simulink model "force_control_sim"  (R2013a)
settings: Solver=FixedStepDiscrete  StartTime=0.0  StopTime=10  FixedStep=.001  RelTol=1e-3
settings Model: Creator=dholley  LastModifiedBy=dholley
settings DataIOCC: LimitDataPoints=off

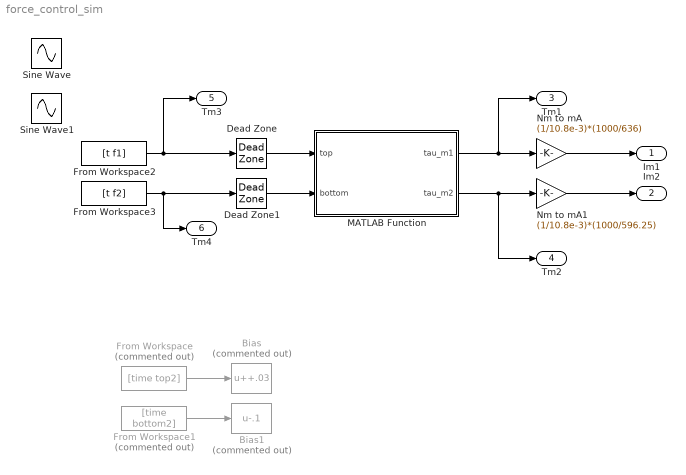
== system force_control_sim ==
  Bias : Bias  Commented=on  Bias=+.03
  Bias1 : Bias  Commented=on  Bias=-.1
  Dead Zone : DeadZone  LowerValue=-.02  UpperValue=.02  SaturateOnIntegerOverflow=on
  Dead Zone1 : DeadZone  LowerValue=-.02  UpperValue=.02  SaturateOnIntegerOverflow=on
  From Workspace : FromWorkspace  Commented=on  VariableName=[time top2]  SampleTime=.001
  From Workspace1 : FromWorkspace  Commented=on  VariableName=[time bottom2]  SampleTime=.001
  From Workspace2 : FromWorkspace  VariableName=[t f1]  SampleTime=0
  From Workspace3 : FromWorkspace  VariableName=[t f2]  SampleTime=0
  MATLAB Function : MATLAB Function  TreatAsAtomicUnit=on
  Nm to mA : Gain  Gain=(1/10.8e-3)*(1000/636)
  Nm to mA1 : Gain  Gain=(1/10.8e-3)*(1000/596.25)
  Sine Wave : Sin  Amplitude=1.7  Frequency=3.14159  SampleTime=0
  Sine Wave1 : Sin  Frequency=3.14159  SampleTime=0
  Im1 : Outport
  Im2 : Outport  Port=2
  Tm1 : Outport  Port=3
  Tm2 : Outport  Port=4
  Tm3 : Outport  Port=5
  Tm4 : Outport  Port=6
  wires:
  MATLAB Function/1(tau_m1) -> Tm1/1, Nm to mA/1
  MATLAB Function/2(tau_m2) -> Tm2/1, Nm to mA1/1
  Nm to mA/1 -> Im1/1
  Nm to mA1/1 -> Im2/1
  Dead Zone1/1 -> MATLAB Function/2(bottom)
  Dead Zone/1 -> MATLAB Function/1(top)
  From Workspace/1 -> Bias/1
  From Workspace1/1 -> Bias1/1
  From Workspace2/1 -> Tm3/1, Dead Zone/1
  From Workspace3/1 -> Tm4/1, Dead Zone1/1

== matlab function force_control_sim/MATLAB Function ==
  data: tau_m1 output; top input; tau_m2 output; bottom input
function [tau_m1,tau_m2] = f2t(top,bottom)
%#codegen

% if top > 0 && bottom > 0 %flexion
% %     mA = (bottom + .171786)/.001822;
%     mA = (bottom + .343572)/.003644;

% elseif top > 0 && bottom < 0
%     mA = (bottom - .120011)/-.001265;
%     mA = (bottom - .240022)/-.00253;

% elseif top < 0 && bottom > 0
%     mA = (bottom + .067092)/-.000959;
%     mA = (bottom + .134184)/-.001918;

% elseif top < 0 && bottom < 0 %extension
% %     mA = (bottom - .075747)/.001458;
%     mA = (bottom - .151494)/.002916;
% 
% else 
%     mA = 0;
%     
        
F1=(top/1901)*(50/.02)*4.4482216;
F2=(bottom/1901)*(50/.02)*4.4482216;

% F2fe=(F1+(.628*F2))/.3157;
% F2ps=F2-F2fe;
% 
% F1fe=-.3123*F2fe;
% F1ps=-.628*F2ps;

% Revision 8/12/14
F1ps=(F1/2.7)-(F2/1.588);
F1fe=(F1+F2)/1.588;
F2ps=(-F1/2.7)+(F2/1.588);
F2fe=(F1+F2)/2.7;


Ffe=((10*F1fe)+(17*F2fe))/27;
Fps=(F1ps-F2ps)/2;

tau_m1=Fps/.76535;
tau_m2=Ffe/.8154;

% if F2fe > 0
%     tau_fe = -.638*F2fe + .3413;
% elseif F2fe < 0
%     tau_fe = -.7058*F2fe - .1488;
% else
%     tau_fe=0;
% end
% 
% if F2ps > 0
%     tau_ps = 1.1639*F2ps - .3562;
% elseif F2ps < 0
%     tau_ps = .9356*F2ps - .4405;
% else
%     tau_ps=0;
% end

% Ffe = (F1 + F2)/2;
% Ffe = (F1/3) + ((2*F2)/3);
% Fps = (F1-F2)/2;

% tau_m2 = (.4279*Fps + 1.8251*Ffe - .00755)/(.54395*.8194);
% tau_m1 = (Fps + 1.9282*Ffe + .1874)/(.41835*1.8866);
% tau_m2 = (1.6738*Fps + 2.9646*Ffe)/(.8936);
% tau_m1 = (Fps + 1.1736*Ffe)/(.25815);


end
